simulink model "Four_Robots_v2"  (R2021a)
settings: Solver=FixedStepAuto  StartTime=0.0  StopTime=t_sim  FixedStep=0.01  RelTol=1e-3  EnableMultiTasking=on
model workspace (MAT data in the model file):
  SL_ROS_VariableLengthArrays_MaxSizes : object (value not decoded)
undefined symbols (not defined in the file or in its folder): Angular, Linear, PP, Way1, Way2, Way3, Way4
libraries: robotlib x16, robotalgslib x8
(part 2 of 2)

== system Four_Robots_v2/TurtleBot4/ Avoiding Obstacles/Path Following ==
  SteeringDirection : Inport
  AngularVelocity : Inport  Port=2
  Action Port : ActionPort  ActionPortLabel=else
  Compute Angular Velocity : MATLAB Function  TreatAsAtomicUnit=on
  Constant : Constant  Value=0
  MaxAngularVelocity : Constant  Value=1.82
  Subtract : Sum  Inputs=+-
  dV : Outport  VectorParamsAs1DForOutWhenUnconnected=off
  dW : Outport  Port=2  VectorParamsAs1DForOutWhenUnconnected=off
  wires:
  Constant/1 -> dV/1
  MaxAngularVelocity/1 -> Compute Angular Velocity/2(wMax)
  SteeringDirection/1 -> Compute Angular Velocity/1(steeringDir)
  Subtract/1 -> dW/1
  Compute Angular Velocity/1(w) -> Subtract/1
  AngularVelocity/1 -> Subtract/2

== system Four_Robots_v2/TurtleBot4/ Avoiding Obstacles/Recovery ==
  LinearVelocity : Inport
  AngularVelocity_comp : Inport  Port=2
  AngularVelocity : Inport  Port=3
  Action Port : ActionPort  ActionPortLabel=if(u1 == 1)
  Gain : Gain  Gain=-1
  Subtract : Sum  Inputs=|+-
  dV : Outport  VectorParamsAs1DForOutWhenUnconnected=off
  dW : Outport  Port=2  VectorParamsAs1DForOutWhenUnconnected=off
  wires:
  AngularVelocity_comp/1 -> Subtract/1
  LinearVelocity/1 -> Gain/1
  Gain/1 -> dV/1
  AngularVelocity/1 -> Subtract/2
  Subtract/1 -> dW/1

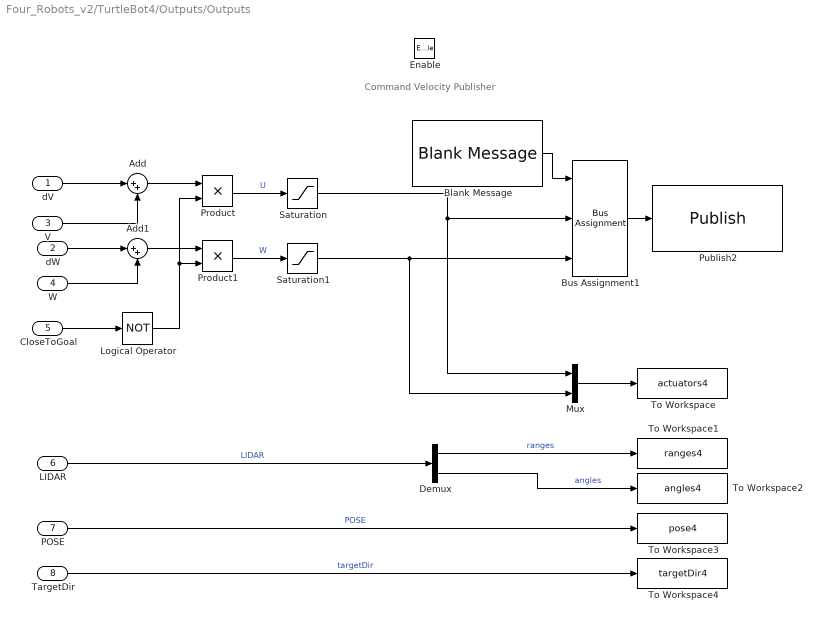
== system Four_Robots_v2/TurtleBot4/Outputs/Outputs ==
  note: Command Velocity Publisher
  dV : Inport
  dW : Inport  Port=2
  V : Inport  Port=3
  W : Inport  Port=4
  CloseToGoal : Inport  Port=5
  LIDAR : Inport  Port=6
  POSE : Inport  Port=7
  TargetDir : Inport  Port=8
  Enable : EnablePort
  Add : Sum  Inputs=|++
  Add1 : Sum  Inputs=|++
  Blank Message : robotlib/Blank Message  messageClass=Message  entityType=geometry_msgs/Twist  messageType=geometry_msgs/Twist  SampleTime=inf  legacyBusStruct=off
  Bus Assignment1 : BusAssignment  DialogController=Simulink.DDGSource_BusAssignment  AssignedSignals=Linear.X,Angular.Z
  Demux : Demux  Outputs=2
  Logical Operator : Logic  Operator=NOT  AllPortsSameDT=off  OutDataTypeStr=boolean
  Mux : Mux  Inputs=2
  Product : Product
  Product1 : Product
  Publish2 : robotlib/Publish  topicSource=Select from ROS network  topic=/robot4/cmd_vel  messageType=geometry_msgs/Twist  legacyBusStruct=off  messageQueueLength=105
  Saturation : Saturate  UpperLimit=PP.DesiredLinearVelocity  LowerLimit=-PP.DesiredLinearVelocity
  Saturation1 : Saturate  UpperLimit=PP.MaxAngularVelocity  LowerLimit=-PP.MaxAngularVelocity
  To Workspace : ToWorkspace  VariableName=actuators4  SaveFormat=Structure With Time  SampleTime=0.01
      settings: Decimation=2
  To Workspace1 : ToWorkspace  VariableName=ranges4  SaveFormat=Structure With Time  SampleTime=0.01
      settings: Decimation=2
  To Workspace2 : ToWorkspace  VariableName=angles4  SaveFormat=Structure With Time  SampleTime=0.01
      settings: Decimation=2
  To Workspace3 : ToWorkspace  VariableName=pose4  SaveFormat=Structure With Time  SampleTime=0.01
      settings: Decimation=2
  To Workspace4 : ToWorkspace  VariableName=targetDir4  SaveFormat=Structure With Time  SampleTime=0.01
      settings: Decimation=2
  wires:
  Demux/1 -> To Workspace1/1  "ranges"
  POSE/1 -> To Workspace3/1  "POSE"
  LIDAR/1 -> Demux/1  "LIDAR"
  Demux/2 -> To Workspace2/1  "angles"
  TargetDir/1 -> To Workspace4/1  "targetDir"
  Saturation1/1 -> Bus Assignment1/3, Mux/2
  Product1/1 -> Saturation1/1  "W"
  Saturation/1 -> Bus Assignment1/2, Mux/1
  Product/1 -> Saturation/1  "U"
  Mux/1 -> To Workspace/1
  Logical Operator/1 -> Product/2, Product1/2
  Bus Assignment1/1 -> Publish2/1
  Blank Message/1 -> Bus Assignment1/1
  Add1/1 -> Product1/1
  Add/1 -> Product/1
  CloseToGoal/1 -> Logical Operator/1
  dW/1 -> Add1/1
  dV/1 -> Add/1
  W/1 -> Add1/2
  V/1 -> Add/2

== matlab function Four_Robots_v2/TurtleBot2/Inputs/MATLAB Function ==
  data: LaserScanMsg input; Ranges output; Angles output
function [Ranges, Angles] = ExtractRangeData(LaserScanMsg)
%#codegen

% Extract Range information
Ranges = double(LaserScanMsg.Ranges);

% Construct Angles vector using AngleMin and AngleIncrement from sensor
% reading.
angMin = double(LaserScanMsg.AngleMin);
angIncrement = double(LaserScanMsg.AngleIncrement);

numReadings = numel(Ranges);
rawAngles = angMin + (0:numReadings-1)' * angIncrement;

% Wrap the angles to the (-pi,pi] interval.
Angles = robotics.internal.wrapToPi(double(rawAngles));

== matlab function Four_Robots_v2/TurtleBot2/Inputs/quad2eul ==
  data: X input; Yaw output; Y input; Z input; W input
function Yaw = quat2eulBlk(X, Y, Z, W)
%#codegen

eularAngles = quat2eul([W, X, Y, Z]);
Yaw = eularAngles(1);

== matlab function Four_Robots_v2/TurtleBot1/ Avoiding Obstacles/Intercollisions ==
  data: i input; dV output; dW output; DATA input; dv_in input; dw_in input; V input; mm output
function [dV,dW,mm] = fcn(i,DATA, dv_in, dw_in, V)
%% DATA
n=4;
POSE1=DATA(1:3);
POSE2=DATA(4:6);
POSE3=DATA(7:9);
POSE4=DATA(10:12);

POSES={POSE1,POSE2,POSE3,POSE4};
POSEi=POSES{i}; %determino el i robot (mismo algoritmo todos los robots)
POSESn={POSEi,POSE2,POSE3,POSE4};

%% Cálculo distancias robots
%di_i no se calcula
% di_2=sqrt((POSEi(1)-POSE2(1))^2+(POSEi(2)-POSE2(2))^2);
d=zeros(1,n-1);
for j=2:n
  POSEj=POSESn{j}; 
  d(j-1)=sqrt((POSEi(1)-POSEj(1))^2+(POSEj(2)-POSEj(2))^2);  
end
%% Test stop
if mod(i,2)==1
    if max(d)<=2.7
        dW = 0;
        dV= -V;
    else
        dW=dw_in;
        dV=dv_in;
    end
else
    dW=dw_in;
    dV=dv_in;
end

mm=max(d)

== matlab function Four_Robots_v2/TurtleBot2/ Avoiding Obstacles/Intercollisions ==
  data: i input; dV output; dW output; DATA input; dv_in input; dw_in input; V input
function [dV,dW] = fcn(i,DATA, dv_in, dw_in, V)
%% DATA
n=4;
POSE1=DATA(1:3);
POSE2=DATA(4:6);
POSE3=DATA(7:9);
POSE4=DATA(10:12);

POSES={POSE1,POSE2,POSE3,POSE4};
POSEi=POSES{i}; %determino el i robot (mismo algoritmo todos los robots)
POSESn={POSEi,POSE1,POSE3,POSE4};

%% Cálculo distancias robots
%di_i no se calcula
% di_2=sqrt((POSEi(1)-POSE2(1))^2+(POSEi(2)-POSE2(2))^2);
d=zeros(1,n-1);
for j=2:n
  POSEj=POSESn{j}; 
  d(j-1)=sqrt((POSEi(1)-POSEj(1))^2+(POSEj(2)-POSEj(2))^2);  
end
%% Test stop
if mod(i,2)==1
    if max(d)<=2.7
        dW = 0;
        dV= -V;
    else
        dW=dw_in;
        dV=dv_in;
    end
else
    dW=dw_in;
    dV=dv_in;
end

== matlab function Four_Robots_v2/TurtleBot4/ Avoiding Obstacles/Intercollisions1 ==
  data: i input; dV output; dW output; DATA input; dv_in input; dw_in input; V input
function [dV,dW] = fcn(i,DATA, dv_in, dw_in, V)
%% DATA
n=4;
POSE1=DATA(1:3);
POSE2=DATA(4:6);
POSE3=DATA(7:9);
POSE4=DATA(10:12);

POSES={POSE1,POSE2,POSE3,POSE4};
POSEi=POSES{i}; %determino el i robot (mismo algoritmo todos los robots)
POSESn={POSEi,POSE1,POSE2,POSE3};

%% Cálculo distancias robots
%di_i no se calcula
% di_2=sqrt((POSEi(1)-POSE2(1))^2+(POSEi(2)-POSE2(2))^2);
d=zeros(1,n-1);
for j=2:n
  POSEj=POSESn{j}; 
  d(j-1)=sqrt((POSEi(1)-POSEj(1))^2+(POSEj(2)-POSEj(2))^2);  
end
%% Test stop
if mod(i,2)==1
    if max(d)<=2.7
        dW = 0;
        dV= -V;
    else
        dW=dw_in;
        dV=dv_in;
    end
else
    dW=dw_in;
    dV=dv_in;
end

== matlab function Four_Robots_v2/TurtleBot4/ Avoiding Obstacles/Path Following/Compute Angular Velocity ==
  data: steeringDir input; w output; wMax input
function w = exampleHelperComputeAngularVelocity(steeringDir, wMax)
%EXAMPLEHELPERCOMPUTEANGULARVELOCITY Compute angular velocity
%   W = exampleHelperComputeAngularVelocity(STEERINGDIR)
%   returns the angular velocity W for a differential drive robot in radians
%   per second for a given steering direction STEERINGDIR in the robot's
%   coordinate frame in radians.
%
%   W = exampleHelperComputeAngularVelocity(STEERINGDIR, WMAX)
%   returns the angular velocity W for a differential drive robot in radians
%   per second for a given steering direction STEERINGDIR in the robot's
%   coordinate frame in radians and maximum angular velocity WMAX in
%   radians per second. The output angular velocity is saturated based on
%   the WMAX.
%
%   Example:
%       
%       w = exampleHelperComputeAngularVelocity(0.2, 1);

% Copyright 2015 The MathWorks, Inc.

%#codegen
%#ok<*EMCA>

% Allow variable input arguments
if nargin == 1   
    wMax = inf;
end

validateattributes(steeringDir, {'double'},{'real'},...
    'exampleHelperComputeAngularVelocity', 'STEERINGDIR', 1);
validateattributes(wMax, {'double'},{'real', 'positive'},...
    'exampleHelperComputeAngularVelocity', 'WMAX', 2);

% Computing in robot's coordinate frame
curPose = [0 0 0];

% The following computation is similar to robotics.PurePursuit
lookaheadPoint = [cos(steeringDir), sin(steeringDir)];
slope = atan2((lookaheadPoint(2) - curPose(2)), ...
    (lookaheadPoint(1) - curPose(1)));
alpha = angdiff(curPose(3), slope);

% Angular velocity command for a differential drive robot is
% equal to the desired curvature to be followed by the robot.

w = (2*sin(alpha));

% Pick a constant rotation when robot is facing in the opposite
% direction of the path
if abs(abs(alpha) - pi) < 1e-12
    w = sign(w)*1;
end

if abs(w) > wMax
    w = sign(w)*wMax;
end

end

== matlab function Four_Robots_v2/TurtleBot4/ Path following/ Extract Goal ==
  data: Waypoints input; Goal output
function Goal = extractGoal(Waypoints)
%#codegen
b = isnan(Waypoints);
[rows,~] = find(b);
ridx = setdiff(1:size(Waypoints,1), sort(rows));
Goal = [Waypoints(ridx(end), 1) Waypoints(ridx(end), 2)];

== matlab function Four_Robots_v2/TurtleBot4/Inputs/MATLAB Function ==
  data: LaserScanMsg input; Ranges output; Angles output
function [Ranges, Angles] = ExtractRangeData(LaserScanMsg)
%#codegen

% Extract Range information
Ranges = double(LaserScanMsg.Ranges);

% Construct Angles vector using AngleMin and AngleIncrement from sensor
% reading.
angMin = double(LaserScanMsg.AngleMin);
angIncrement = double(LaserScanMsg.AngleIncrement);

numReadings = numel(Ranges);
rawAngles = angMin + (0:numReadings-1)' * angIncrement;

% Wrap the angles to the (-pi,pi] interval.
Angles = robotics.internal.wrapToPi(double(rawAngles));

== matlab function Four_Robots_v2/TurtleBot4/Inputs/quad2eul ==
  data: X input; Yaw output; Y input; Z input; W input
function Yaw = quat2eulBlk(X, Y, Z, W)
%#codegen

eularAngles = quat2eul([W, X, Y, Z]);
Yaw = eularAngles(1);

== matlab function Four_Robots_v2/TurtleBot3/ Avoiding Obstacles/Intercollisions1 ==
  data: i input; dV output; dW output; DATA input; dv_in input; dw_in input; V input
function [dV,dW] = fcn(i,DATA, dv_in, dw_in, V)
%% DATA
n=4;
POSE1=DATA(1:3);
POSE2=DATA(4:6);
POSE3=DATA(7:9);
POSE4=DATA(10:12);

POSES={POSE1,POSE2,POSE3,POSE4};
POSEi=POSES{i}; %determino el i robot (mismo algoritmo todos los robots)
POSESn={POSEi,POSE1,POSE2,POSE4};

%% Cálculo distancias robots
%di_i no se calcula
% di_2=sqrt((POSEi(1)-POSE2(1))^2+(POSEi(2)-POSE2(2))^2);
d=zeros(1,n-1);
for j=2:n
  POSEj=POSESn{j}; 
  d(j-1)=sqrt((POSEi(1)-POSEj(1))^2+(POSEj(2)-POSEj(2))^2);  
end
%% Test stop
if mod(i,2)==1
    if max(d)<=2.7
        dW = 0;
        dV= -V;
    else
        dW=dw_in;
        dV=dv_in;
    end
else
    dW=dw_in;
    dV=dv_in;
end

== matlab function Four_Robots_v2/TurtleBot3/ Avoiding Obstacles/Path Following/Compute Angular Velocity ==
  data: steeringDir input; w output; wMax input
function w = exampleHelperComputeAngularVelocity(steeringDir, wMax)
%EXAMPLEHELPERCOMPUTEANGULARVELOCITY Compute angular velocity
%   W = exampleHelperComputeAngularVelocity(STEERINGDIR)
%   returns the angular velocity W for a differential drive robot in radians
%   per second for a given steering direction STEERINGDIR in the robot's
%   coordinate frame in radians.
%
%   W = exampleHelperComputeAngularVelocity(STEERINGDIR, WMAX)
%   returns the angular velocity W for a differential drive robot in radians
%   per second for a given steering direction STEERINGDIR in the robot's
%   coordinate frame in radians and maximum angular velocity WMAX in
%   radians per second. The output angular velocity is saturated based on
%   the WMAX.
%
%   Example:
%       
%       w = exampleHelperComputeAngularVelocity(0.2, 1);

% Copyright 2015 The MathWorks, Inc.

%#codegen
%#ok<*EMCA>

% Allow variable input arguments
if nargin == 1   
    wMax = inf;
end

validateattributes(steeringDir, {'double'},{'real'},...
    'exampleHelperComputeAngularVelocity', 'STEERINGDIR', 1);
validateattributes(wMax, {'double'},{'real', 'positive'},...
    'exampleHelperComputeAngularVelocity', 'WMAX', 2);

% Computing in robot's coordinate frame
curPose = [0 0 0];

% The following computation is similar to robotics.PurePursuit
lookaheadPoint = [cos(steeringDir), sin(steeringDir)];
slope = atan2((lookaheadPoint(2) - curPose(2)), ...
    (lookaheadPoint(1) - curPose(1)));
alpha = angdiff(curPose(3), slope);

% Angular velocity command for a differential drive robot is
% equal to the desired curvature to be followed by the robot.

w = (2*sin(alpha));

% Pick a constant rotation when robot is facing in the opposite
% direction of the path
if abs(abs(alpha) - pi) < 1e-12
    w = sign(w)*1;
end

if abs(w) > wMax
    w = sign(w)*wMax;
end

end

== matlab function Four_Robots_v2/TurtleBot3/ Path following/ Extract Goal ==
  data: Waypoints input; Goal output
function Goal = extractGoal(Waypoints)
%#codegen
b = isnan(Waypoints);
[rows,~] = find(b);
ridx = setdiff(1:size(Waypoints,1), sort(rows));
Goal = [Waypoints(ridx(end), 1) Waypoints(ridx(end), 2)];

== matlab function Four_Robots_v2/TurtleBot1/ Avoiding Obstacles/Path Following/Compute Angular Velocity ==
  data: steeringDir input; w output; wMax input
function w = exampleHelperComputeAngularVelocity(steeringDir, wMax)
%EXAMPLEHELPERCOMPUTEANGULARVELOCITY Compute angular velocity
%   W = exampleHelperComputeAngularVelocity(STEERINGDIR)
%   returns the angular velocity W for a differential drive robot in radians
%   per second for a given steering direction STEERINGDIR in the robot's
%   coordinate frame in radians.
%
%   W = exampleHelperComputeAngularVelocity(STEERINGDIR, WMAX)
%   returns the angular velocity W for a differential drive robot in radians
%   per second for a given steering direction STEERINGDIR in the robot's
%   coordinate frame in radians and maximum angular velocity WMAX in
%   radians per second. The output angular velocity is saturated based on
%   the WMAX.
%
%   Example:
%       
%       w = exampleHelperComputeAngularVelocity(0.2, 1);

% Copyright 2015 The MathWorks, Inc.

%#codegen
%#ok<*EMCA>

% Allow variable input arguments
if nargin == 1   
    wMax = inf;
end

validateattributes(steeringDir, {'double'},{'real'},...
    'exampleHelperComputeAngularVelocity', 'STEERINGDIR', 1);
validateattributes(wMax, {'double'},{'real', 'positive'},...
    'exampleHelperComputeAngularVelocity', 'WMAX', 2);

% Computing in robot's coordinate frame
curPose = [0 0 0];

% The following computation is similar to robotics.PurePursuit
lookaheadPoint = [cos(steeringDir), sin(steeringDir)];
slope = atan2((lookaheadPoint(2) - curPose(2)), ...
    (lookaheadPoint(1) - curPose(1)));
alpha = angdiff(curPose(3), slope);

% Angular velocity command for a differential drive robot is
% equal to the desired curvature to be followed by the robot.

w = (2*sin(alpha));

% Pick a constant rotation when robot is facing in the opposite
% direction of the path
if abs(abs(alpha) - pi) < 1e-12
    w = sign(w)*1;
end

if abs(w) > wMax
    w = sign(w)*wMax;
end

end

== matlab function Four_Robots_v2/TurtleBot1/ Path following/ Extract Goal ==
  data: Waypoints input; Goal output
function Goal = extractGoal(Waypoints)
%#codegen
b = isnan(Waypoints);
[rows,~] = find(b);
ridx = setdiff(1:size(Waypoints,1), sort(rows));
Goal = [Waypoints(ridx(end), 1) Waypoints(ridx(end), 2)];

== matlab function Four_Robots_v2/TurtleBot2/ Avoiding Obstacles/Path Following/Compute Angular Velocity ==
  data: steeringDir input; w output; wMax input
function w = exampleHelperComputeAngularVelocity(steeringDir, wMax)
%EXAMPLEHELPERCOMPUTEANGULARVELOCITY Compute angular velocity
%   W = exampleHelperComputeAngularVelocity(STEERINGDIR)
%   returns the angular velocity W for a differential drive robot in radians
%   per second for a given steering direction STEERINGDIR in the robot's
%   coordinate frame in radians.
%
%   W = exampleHelperComputeAngularVelocity(STEERINGDIR, WMAX)
%   returns the angular velocity W for a differential drive robot in radians
%   per second for a given steering direction STEERINGDIR in the robot's
%   coordinate frame in radians and maximum angular velocity WMAX in
%   radians per second. The output angular velocity is saturated based on
%   the WMAX.
%
%   Example:
%       
%       w = exampleHelperComputeAngularVelocity(0.2, 1);

% Copyright 2015 The MathWorks, Inc.

%#codegen
%#ok<*EMCA>

% Allow variable input arguments
if nargin == 1   
    wMax = inf;
end

validateattributes(steeringDir, {'double'},{'real'},...
    'exampleHelperComputeAngularVelocity', 'STEERINGDIR', 1);
validateattributes(wMax, {'double'},{'real', 'positive'},...
    'exampleHelperComputeAngularVelocity', 'WMAX', 2);

% Computing in robot's coordinate frame
curPose = [0 0 0];

% The following computation is similar to robotics.PurePursuit
lookaheadPoint = [cos(steeringDir), sin(steeringDir)];
slope = atan2((lookaheadPoint(2) - curPose(2)), ...
    (lookaheadPoint(1) - curPose(1)));
alpha = angdiff(curPose(3), slope);

% Angular velocity command for a differential drive robot is
% equal to the desired curvature to be followed by the robot.

w = (2*sin(alpha));

% Pick a constant rotation when robot is facing in the opposite
% direction of the path
if abs(abs(alpha) - pi) < 1e-12
    w = sign(w)*1;
end

if abs(w) > wMax
    w = sign(w)*wMax;
end

end

== matlab function Four_Robots_v2/TurtleBot1/Inputs/MATLAB Function ==
  data: LaserScanMsg input; Ranges output; Angles output
function [Ranges, Angles] = ExtractRangeData(LaserScanMsg)
%#codegen

% Extract Range information
Ranges = double(LaserScanMsg.Ranges);

% Construct Angles vector using AngleMin and AngleIncrement from sensor
% reading.
angMin = double(LaserScanMsg.AngleMin);
angIncrement = double(LaserScanMsg.AngleIncrement);

numReadings = numel(Ranges);
rawAngles = angMin + (0:numReadings-1)' * angIncrement;

% Wrap the angles to the (-pi,pi] interval.
Angles = robotics.internal.wrapToPi(double(rawAngles));

== matlab function Four_Robots_v2/TurtleBot3/Inputs/MATLAB Function ==
  data: LaserScanMsg input; Ranges output; Angles output
function [Ranges, Angles] = ExtractRangeData(LaserScanMsg)
%#codegen

% Extract Range information
Ranges = double(LaserScanMsg.Ranges);

% Construct Angles vector using AngleMin and AngleIncrement from sensor
% reading.
angMin = double(LaserScanMsg.AngleMin);
angIncrement = double(LaserScanMsg.AngleIncrement);

numReadings = numel(Ranges);
rawAngles = angMin + (0:numReadings-1)' * angIncrement;

% Wrap the angles to the (-pi,pi] interval.
Angles = robotics.internal.wrapToPi(double(rawAngles));

== matlab function Four_Robots_v2/TurtleBot1/Inputs/quad2eul ==
  data: X input; Yaw output; Y input; Z input; W input
function Yaw = quat2eulBlk(X, Y, Z, W)
%#codegen

eularAngles = quat2eul([W, X, Y, Z]);
Yaw = eularAngles(1);

== matlab function Four_Robots_v2/TurtleBot3/Inputs/quad2eul ==
  data: X input; Yaw output; Y input; Z input; W input
function Yaw = quat2eulBlk(X, Y, Z, W)
%#codegen

eularAngles = quat2eul([W, X, Y, Z]);
Yaw = eularAngles(1);

== matlab function Four_Robots_v2/TurtleBot2/ Path following/ Extract Goal ==
  data: Waypoints input; Goal output
function Goal = extractGoal(Waypoints)
%#codegen
b = isnan(Waypoints);
[rows,~] = find(b);
ridx = setdiff(1:size(Waypoints,1), sort(rows));
Goal = [Waypoints(ridx(end), 1) Waypoints(ridx(end), 2)];
